simulink model "TP4_Simulink"  (R2018b)
settings: Solver=VariableStepAuto  StartTime=0.0  StopTime=10.0  RelTol=1e-3
values from neighbouring files (symbols this model uses):
  C1 = 1    [TP4_MatlabUnitario.m]    (also in TP4_MatlabValores.m)
undefined symbols (not defined in the file or in its folder): s
settings Model: Creator=A47521  LastModifiedBy=A47521

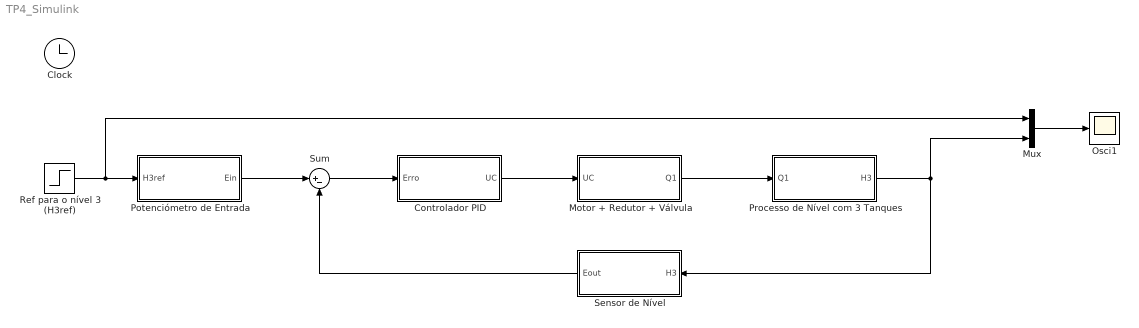
== system TP4_Simulink ==
  Clock : Clock
  Controlador PID : Subsystem
  Motor + Redutor + Válvula : Subsystem
  Mux : Mux  Inputs=2
  Osci1 : Scope
  Potenciómetro de Entrada : Subsystem
  Processo de Nível com 3 Tanques : Subsystem
  Ref para o nível 3 (H3ref) : Step  SampleTime=0
  Sensor de Nível : Subsystem
  Sum : Sum  Inputs=|+-
  wires:
  Controlador PID/1(UC) -> Motor + Redutor + Válvula/1(UC)
  Motor + Redutor + Válvula/1(Q1) -> Processo de Nível com 3 Tanques/1(Q1)
  Processo de Nível com 3 Tanques/1(H3) -> Mux/2, Sensor de Nível/1(H3)
  Sensor de Nível/1(Eout) -> Sum/2
  Potenciómetro de Entrada/1(Ein) -> Sum/1
  Sum/1 -> Controlador PID/1(Erro)
  Ref para o nível 3 (H3ref)/1 -> Mux/1, Potenciómetro de Entrada/1(H3ref)
  Mux/1 -> Osci1/1

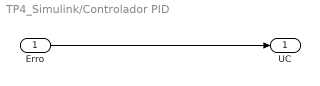
== system TP4_Simulink/Controlador PID ==
  Erro : Inport
  UC : Outport
  wires:
  Erro/1 -> UC/1

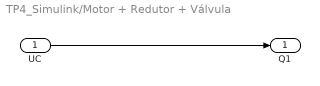
== system TP4_Simulink/Motor + Redutor + Válvula ==
  UC : Inport
  Q1 : Outport
  wires:
  UC/1 -> Q1/1

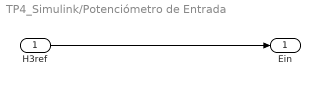
== system TP4_Simulink/Potenciómetro de Entrada ==
  H3ref : Inport
  Ein : Outport
  wires:
  H3ref/1 -> Ein/1

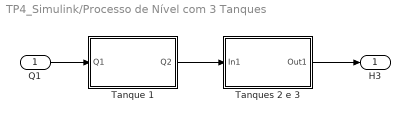
== system TP4_Simulink/Processo de Nível com 3 Tanques ==
  Q1 : Inport
  Tanque 1 : Subsystem
  Tanques 2 e 3 : Subsystem
  H3 : Outport
  wires:
  Q1/1 -> Tanque 1/1(Q1)
  Tanque 1/1(Q2) -> Tanques 2 e 3/1(In1)
  Tanques 2 e 3/1(Out1) -> H3/1

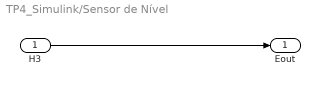
== system TP4_Simulink/Sensor de Nível ==
  H3 : Inport
  Eout : Outport
  wires:
  H3/1 -> Eout/1

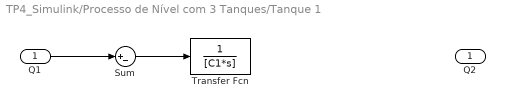
== system TP4_Simulink/Processo de Nível com 3 Tanques/Tanque 1 ==
  Q1 : Inport
  Sum : Sum  Inputs=|+-
  Transfer Fcn : TransferFcn  Denominator=[C1*s]
  Q2 : Outport
  wires:
  Q1/1 -> Sum/1
  Sum/1 -> Transfer Fcn/1

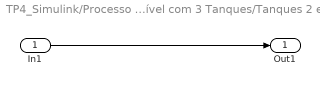
== system TP4_Simulink/Processo de Nível com 3 Tanques/Tanques 2 e 3 ==
  In1 : Inport
  Out1 : Outport
  wires:
  In1/1 -> Out1/1
